simulink model "basicFeedbackSystem_discrete"  (R2019b)
settings: Solver=VariableStepAuto  StartTime=0.0  StopTime=10.0  RelTol=1e-3
libraries: dspsigops x2
settings Model: Creator=23731  LastModifiedBy=23731

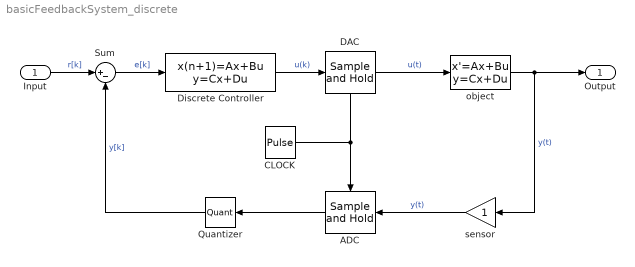
== system basicFeedbackSystem_discrete ==
  Input : Inport
  ADC : dspsigops/Sample and Hold  trig=Rising edge  initCond=0  latchinput=off
  CLOCK : DiscretePulseGenerator  PulseType=Time based  Period=10  PulseWidth=5
  DAC : dspsigops/Sample and Hold  trig=Rising edge  initCond=0  latchinput=off
  Discrete Controller : DiscreteStateSpace  SampleTime=-1
  Quantizer : Quantizer  QuantizationInterval=0.001
  Sum : Sum  Inputs=|+-
  object : StateSpace  InitialCondition=0
  sensor : Gain
  Output : Outport
  wires:
  Input/1 -> Sum/1  "r[k]"
  Sum/1 -> Discrete Controller/1  "e[k]"
  object/1 -> Output/1, sensor/1  "y(t)"
  Quantizer/1 -> Sum/2  "y[k]"
  Discrete Controller/1 -> DAC/1  "u(k)"
  DAC/1 -> object/1  "u(t)"
  sensor/1 -> ADC/1  "y(t)"
  ADC/1 -> Quantizer/1
  CLOCK/1 -> DAC/Trigger, ADC/Trigger
